simulink model "hp_val"  (R2024a)
settings: Solver=VariableStepAuto  StartTime=0.0  StopTime=0.1  MaxStep=1e-4  RelTol=1e-4  AbsTol=1e-3
values from neighbouring files (symbols this model uses):
  base = hexapod.base    [calcMotorAngles.m]    (also in calcMotorAngles2.m; calcMotorAngles3.m; calcQ.m; calcQ2_bak.m)
  coupler = hexapod.coupler    [calcMotorAngles.m]    (also in calcMotorAngles2.m; calcMotorAngles3.m; calcQ.m; calcQ2_bak.m)
  excenter = hexapod.excenter    [calcMotorAngles.m]    (also in calcMotorAngles2.m; calcMotorAngles3.m; calcQ.m; calcQ2_bak.m)
  N = size(M, 1)    [generateMotorDataFromFile.m]    (also in generateMotorDataFromTrajFile.m; main.m = 9; main_feedforward.m = 36; rw.m = size(data, 1))
  platform = hexapod.platform    [calcMotorAngles.m]    (also in calcMotorAngles2.m; calcMotorAngles3.m; calcQ.m; calcQ2_bak.m)
  q = q_rots    [q_test.m]
  Y = fft(motorAnglesmask(:, col))    [calc_spring_param.m]
undefined symbols (not defined in the file or in its folder): X, y_zero, Z
libraries: sm_lib x59, nesl_utility x37
(part 1 of 3)
settings Model: Creator=james  LastModifiedBy=james
settings ExplorerConfigSet: InternalSimMechanicsExplorerSettings="<ExplorerConfiguration><canonicalview>planar_xy</canonicalview><AnimationSetting><BasePlaybackSpeed>1.0</BasePlaybackSpeed><PlaybackSpeedFactor>1.0</PlaybackSpeedFactor></AnimationSetting><TilePanel><TileInfo><Tiles Columns=\"1\" Count=\"1\" Rows=\"1\"><Column Weight=\"1\"/><Row Weight=\"1\"/><Tile Height=\"1\" Width=\"1\" X=\"0\" Y=\"0\"/></Tiles></TileInfo><SceneInfo><SceneViewer><BGColor><R>0.60000002384185791</R><G>0.60000002384185791</G><B>0.60000002384185791</B></BGColor><Camera><DoPerspective>off</DoPerspective><Position><X>0.407634035868538969</X><Y>0.593101480541867065</Y><Z>0.669480552198040701</Z></Position><Center><X>0.0276287287639288004</X><Y>-0.0490949755488107042</Y><Z>0.00376313590377908014</Z></Center><Up><X>-0.546669275478287031</X><Y>0.73648910450049665</Y><Z>-0.398417497356859773</Z></Up><ViewLimDist>1</ViewLimDist><YLim>0.355880954265594518</YLim><XLim>0.467563920400976163</XLim></Camera></SceneViewer></SceneInfo></TilePanel><MechEditorPanel><Cameras/><GfxPanelCameraMap/><VideoCreator><PlaybackSpeedRatio>1.0</PlaybackSpeedRatio><FrameRate>30</FrameRate><VideoFormat>Motion JPEG AVI</VideoFormat><FrameSize>auto</FrameSize></VideoCreator></MechEditorPanel></ExplorerConfiguration>"

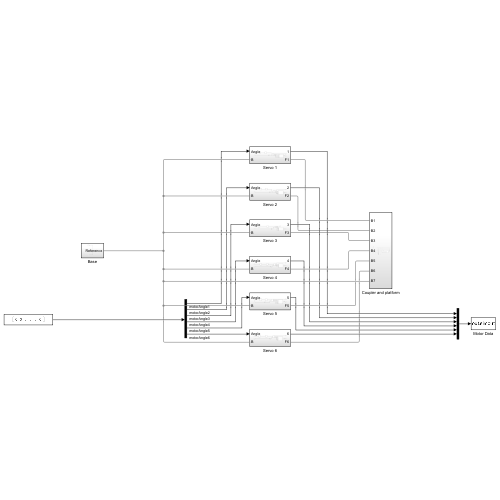
[thumbnail: Simulink's stored preview of the top-level diagram]
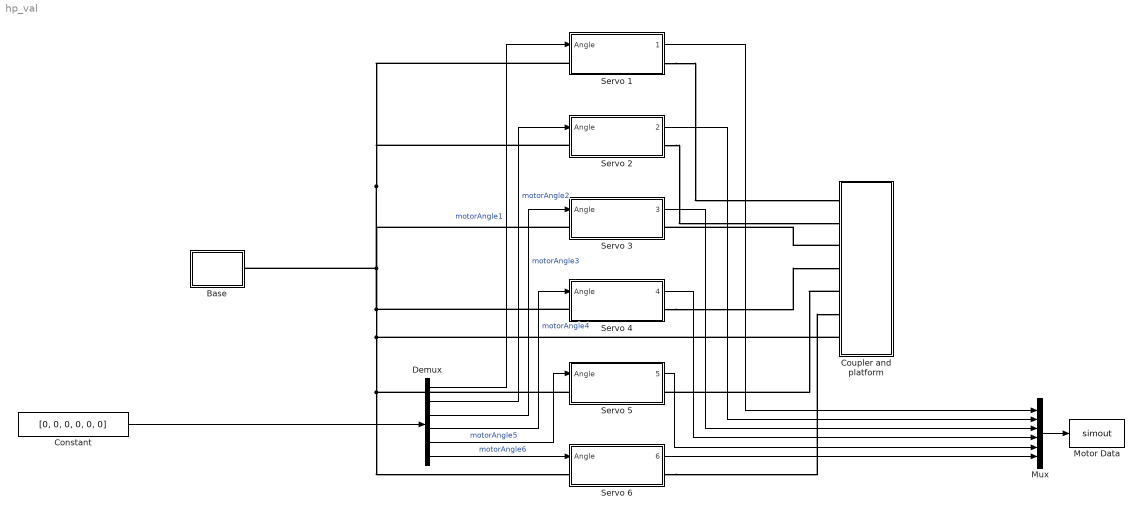
== system hp_val ==
  Base : Subsystem
  Constant : Constant  Value=[0, 0, 0, 0, 0, 0]
  Coupler and platform : Subsystem
  Demux : Demux  Outputs=6
  Motor Data : ToWorkspace  VariableName=simout  SaveFormat=Timeseries  SampleTime=-1
  Mux : Mux  Inputs=6
  Servo 1 : Subsystem
  Servo 2 : Subsystem
  Servo 3 : Subsystem
  Servo 4 : Subsystem
  Servo 5 : Subsystem
  Servo 6 : Subsystem
  wires:
  Constant/1 -> Demux/1
  Demux/3 -> Servo 3/1(Angle)  "motorAngle3"
  Mux/1 -> Motor Data/1
  Servo 6/1(6) -> Mux/6
  Demux/2 -> Servo 2/1(Angle)  "motorAngle2"
  Demux/5 -> Servo 5/1(Angle)  "motorAngle5"
  Demux/4 -> Servo 4/1(Angle)  "motorAngle4"
  Servo 4/1(4) -> Mux/4
  Servo 1/1(1) -> Mux/1
  Demux/1 -> Servo 1/1(Angle)  "motorAngle1"
  Servo 3/1(3) -> Mux/3
  Demux/6 -> Servo 6/1(Angle)  "motorAngle6"
  Servo 2/1(2) -> Mux/2
  Servo 5/1(5) -> Mux/5
  connections:
  Servo 4/LConn1 -- Servo 1/LConn1 -- Servo 2/LConn1 -- Servo 3/LConn1 -- Base/RConn1 -- Coupler and platform/LConn7 -- Servo 5/LConn1 -- Servo 6/LConn1
  Coupler and platform/LConn5 -- Servo 5/RConn1
  Servo 4/RConn1 -- Coupler and platform/LConn4
  Servo 1/RConn1 -- Coupler and platform/LConn1
  Coupler and platform/LConn3 -- Servo 3/RConn1
  Servo 6/RConn1 -- Coupler and platform/LConn6
  Servo 2/RConn1 -- Coupler and platform/LConn2

== system hp_val/Base ==
  Mechanism Configuration : sm_lib/Utilities/Mechanism Configuration  UniformGravity=Constant  GravityVector=[0 -9.80665 0]  GravityVectorUnits=m/s^2  LinearizationDelta=0.001  JointModeTransitionNonlinearIterations=2
  Solver Configuration : nesl_utility/Solver Configuration  PhysicalDomain=network_engine_domain  SubClassName=solver  LeftPortType=input  RightPortType=generic  Tones=[]  Harmonics=[]  SimulateNoise=off  Profile=off  UseLocalSampling=off  EnableSwitchedLinearOptims=on  FrequencyDomain=off  UseCCode=off  RelTol=0.001  AbsTol=1e-06  MinStep=1e-09  ToWorkspace=off  RevertToSquareIcSolve=off  NumHomotopyIterations=100  PhasorMode=off  PhasorModeNumHarmonics=1  ConsistencySolver=NEWTON_XTOL_AFTER_FTOL  IndexReductionMethod=DerivativeReplacement  DoDC=off  ResidualTolerance=1e-09  ConsistencyTolSource=GLOBAL  ConsistencyAbsTol=0.001  ConsistencyRelTol=0.001  ConsistencyTolFactor=0.001  UseLocalSolver=off  LocalSolverChoice=NE_BACKWARD_EULER_ADVANCER  ResolveIndetEquations=on  FunctionEvalNumThread=1  LocalSolverSampleTime=0.001  DoFixedCost=off  MaxNonlinIter=3  MaxModeIter=2  ComputeImpulses=off  ImpulseIterations=2  LinearAlgebra=Sparse  LinearAlgebraNumThread=0  EquationFormulation=NE_TIME_EF  DelaysMemoryBudget=1024  AutomaticFiltering=on  FilteringTimeConstant=0.001  PartitionStorageMethod=AS_NEEDED  PartitionMemoryBudget=1024  PartitionMethod=FAST  MultibodyUseLocalSolver=off  MultibodyLocalSolverChoice=ODE1  MultibodyLocalSolverSampleTime=0.001
  World Frame : sm_lib/Frames and Transforms/World Frame
  Reference : PMIOPort  Side=Right
  connections:
  World Frame/RConn1 -- Reference/RConn1 -- Mechanism Configuration/RConn1 -- Solver Configuration/RConn1
